simulink model "wwec_rlONEbody2"  (R2017b)
settings: Solver=VariableStepAuto  StartTime=0.0  StopTime=tsim  RelTol=1e-3
values from neighbouring files (symbols this model uses):
  A1 = 3.3e5    (= 330000)    [CS533DQN_FunctionApproximation.m]    (also in ContinousControl.m; DeepQLearningF.m; EtanStateExtraction.m; HopeGreatRLCode.m)
  B1 = 9.7e4    (= 97000)    [CS533DQN_FunctionApproximation.m]    (also in ContinousControl.m; DeepQLearningF.m; EtanStateExtraction.m = 450000; HopeGreatRLCode.m)
  B2 = action(action_idx,1)    [CS533DQN_FunctionApproximation.m]    (also in ContinousControl.m; DeepQLearningF.m; EtanStateExtraction.m = B2Matrix(1,b); HopeGreatRLCode.m = 0)
  K1 = 8.8e5    (= 880000)    [CS533DQN_FunctionApproximation.m]    (also in ContinousControl.m; DeepQLearningF.m; EtanStateExtraction.m = 6000000; HopeGreatRLCode.m)
  K2 = action(action_idx,2)    [CS533DQN_FunctionApproximation.m]    (also in ContinousControl.m; DeepQLearningF.m; EtanStateExtraction.m = K2Matrix(1,Ck); HopeGreatRLCode.m = 0)
  m1 = 9.7e4    (= 97000)    [CS533DQN_FunctionApproximation.m]    (also in ContinousControl.m; DeepQLearningF.m; EtanStateExtraction.m; HopeGreatRLCode.m)
settings Model: Creator=brekken  LastModifiedBy=ghorbanl
settings CodeAppCC: StateflowObjectComments=on

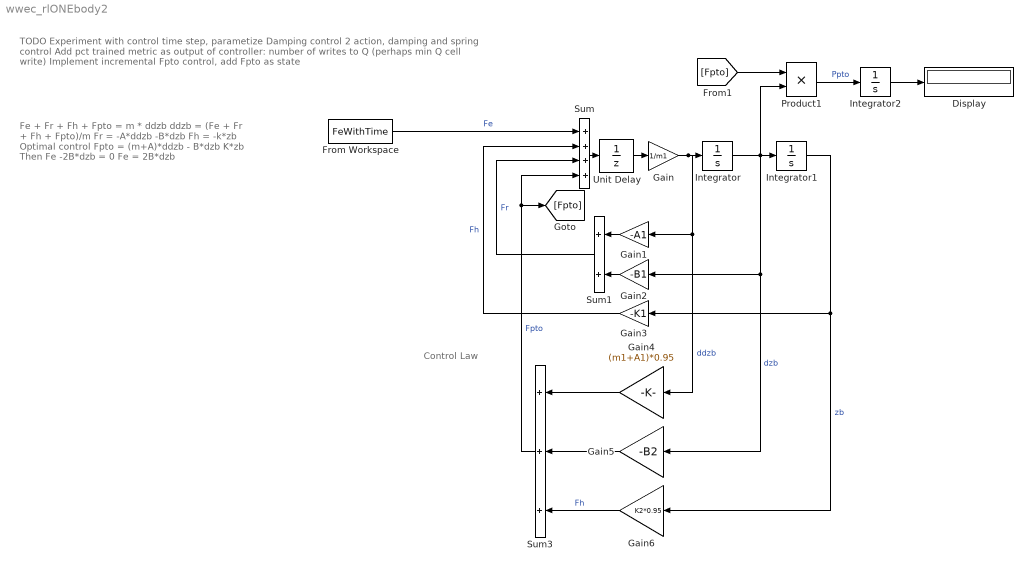
== system wwec_rlONEbody2 ==
  note: Control Law
  note: TODO
      |
      | Experiment with control time step, parametize
      | Damping control
      | 2 action, damping and spring control
      | Add pct trained metric as output of controller: number of writes to Q (perhaps min Q cell write)
      | Implement incremental Fpto control, add Fpto as state
  note: Fe + Fr + Fh + Fpto = m * ddzb
      | ddzb = (Fe + Fr + Fh + Fpto)/m
      |
      | Fr = -A*ddzb -B*dzb
      |
      | Fh = -k*zb
      |
      | Optimal control
      | Fpto = (m+A)*ddzb - B*dzb K*zb
      | Then
      | Fe -2B*dzb = 0
      | Fe = 2B*dzb
  Display : Display
  From Workspace : FromWorkspace  VariableName=FeWithTime  SampleTime=0  OutputAfterFinalValue=Setting to zero
  Gain : Gain  Gain=1/m1
  Gain1 : Gain  Gain=-A1
  Gain2 : Gain  Gain=-B1
  Gain3 : Gain  Gain=-K1
  Gain4 : Gain  Gain=(m1+A1)*0.95
  Gain5 : Gain  Gain=-B2
  Gain6 : Gain  Gain=K2*0.95
  Integrator : Integrator
  Integrator1 : Integrator
  Integrator2 : Integrator
  Product1 : Product
  Sum : Sum  Inputs=++++
  Sum1 : Sum
  Sum3 : Sum  Inputs=+++
  Unit Delay : UnitDelay  SampleTime=-1
  wires:
  Gain/1 -> Gain1/1, Gain4/1, Integrator/1  "ddzb"
  Sum1/1 -> Sum/3  "Fr"
  Gain3/1 -> Sum/2  "Fh"
  Gain1/1 -> Sum1/1
  Gain2/1 -> Sum1/2
  From Workspace/1 -> Sum/1  "Fe"
  Product1/1 -> Integrator2/1  "Ppto"
  Integrator2/1 -> Display/1
  [Fpto] -> Product1/1
  Integrator1/1 -> Gain6/1, Gain3/1  "zb"
  Gain5/1 -> Sum3/2
  Integrator/1 -> Product1/2, Gain5/1, Gain2/1, Integrator1/1  "dzb"
  Gain4/1 -> Sum3/1
  Gain6/1 -> Sum3/3  "Fh"
  Sum3/1 -> [Fpto], Sum/4  "Fpto"
  Sum/1 -> Unit Delay/1
  Unit Delay/1 -> Gain/1
